simulink model "Subsystem"  (R2020b)
settings: Solver=FixedStepAuto  StartTime=0.0  StopTime=10.0  FixedStep=0.2  RelTol=1e-3
values from neighbouring files (symbols this model uses):
  a0 = 1.0    [data_dict.sldd]
  a1 = -2.0    [data_dict.sldd]
  a2 = -1.0    [data_dict.sldd]
  a3 = 1.0    [data_dict.sldd]
  a4 = 1.0    [data_dict.sldd]
  a5 = -1.0    [data_dict.sldd]
settings Model: DataDictionary=data_dict.sldd  Creator=Shree  LastModifiedBy=Shree
settings DataIOCC: SaveOutput=off  SaveTime=off

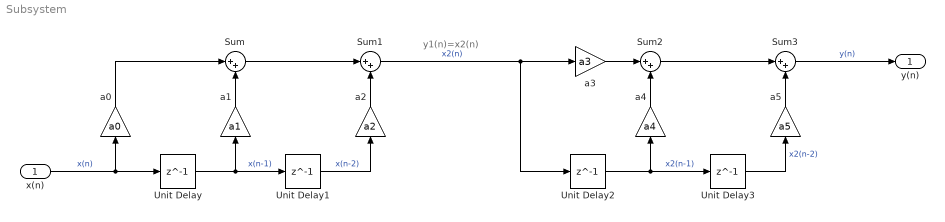
== system Subsystem ==
  note: y1(n)=x2(n)
  x(n) : Inport  OutDataTypeStr=double  PortDimensions=1  SampleTime=[0.20000000000000001,0]
  Sum{,1..3} (4 alike) : Sum  Inputs=|++
  Unit Delay{,1..3} (4 alike) : Delay  DelayLength=1  InitialCondition=0
  a0 : Gain  Gain=a0
  a1 : Gain  Gain=a1
  a2 : Gain  Gain=a2
  a3 : Gain  Gain=a3
  a4 : Gain  Gain=a4
  a5 : Gain  Gain=a5
  y(n) : Outport  OutDataTypeStr=double  PortDimensions=1  SampleTime=[0.20000000000000001,0]
  wires:
  Unit Delay/1 -> Unit Delay1/1, a1/1  "x(n-1)"
  Sum2/1 -> Sum3/1
  Sum1/1 -> Unit Delay2/1, a3/1  "x2(n)"
  Unit Delay1/1 -> a2/1  "x(n-2)"
  Sum/1 -> Sum1/1
  a2/1 -> Sum1/2
  x(n)/1 -> a0/1, Unit Delay/1  "x(n)"
  a4/1 -> Sum2/2
  a5/1 -> Sum3/2
  Unit Delay3/1 -> a5/1  "x2(n-2)"
  Unit Delay2/1 -> Unit Delay3/1, a4/1  "x2(n-1)"
  a1/1 -> Sum/2
  a0/1 -> Sum/1
  a3/1 -> Sum2/1
  Sum3/1 -> y(n)/1  "y(n)"
